simulink model "controller"  (R2021b)
settings: Solver=FixedStepAuto  StartTime=0.0  StopTime=10.0  RelTol=1e-3
settings Model: Creator=lywan  LastModifiedBy=lywan
settings OptimizationCC: ZeroExternalMemoryAtStartup=off  ZeroInternalMemoryAtStartup=off
settings RTWCC: GenCodeOnly=on  Toolchain=AUTOSAR Adaptive | CMake  TargetLang=C++
settings GRTTargetCC: TargetLangStandard=C++11 (ISO)  CodeInterfacePackaging=C++ class  MultiInstanceErrorCode=None

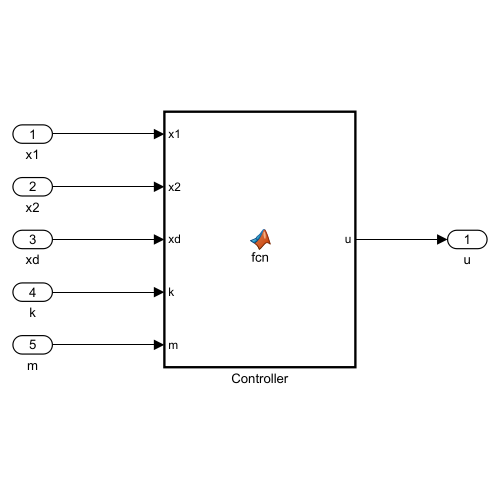
[thumbnail: Simulink's stored preview of the top-level diagram]
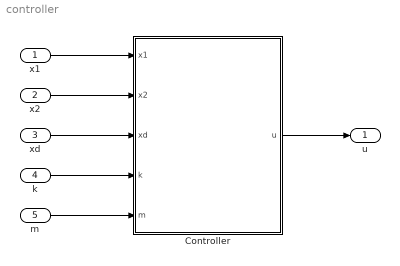
== system controller ==
  x1 : Inport
  x2 : Inport  Port=2
  xd : Inport  Port=3
  k : Inport  Port=4
  m : Inport  Port=5
  Controller : MATLAB Function  TreatAsAtomicUnit=on
  u : Outport
  wires:
  x1/1 -> Controller/1(x1)
  x2/1 -> Controller/2(x2)
  xd/1 -> Controller/3(xd)
  k/1 -> Controller/4(k)
  m/1 -> Controller/5(m)
  Controller/1(u) -> u/1

== matlab function controller/Controller ==
  data: x1 input; u output; x2 input; xd input; k input; m input
function u = fcn(x1, x2, xd, k, m)

e = xd - x1;
k1 = -m + k;
k2 = 2*m;
% k1 = -100*m + k;
% k2 = 20*m;
u = -k1*e - k2*x2 + k*xd;

%% LQR at m = 10, k = 2, Q = [100, 0; 0, 0.01], R = 0.001
% e = xd - x1;
% % k1 = -12.2829;
% % k2 = 15.9893;
% k1 = -314.2341;
% k2 = 79.3390;
% u = -k1*e - k2*x2 + k*xd;
